simulink model "EXP1"  (R2020b)
settings: Solver=VariableStepAuto  StartTime=0.0  StopTime=200  RelTol=1e-3
settings Model: Creator=dssan  LastModifiedBy=dssan

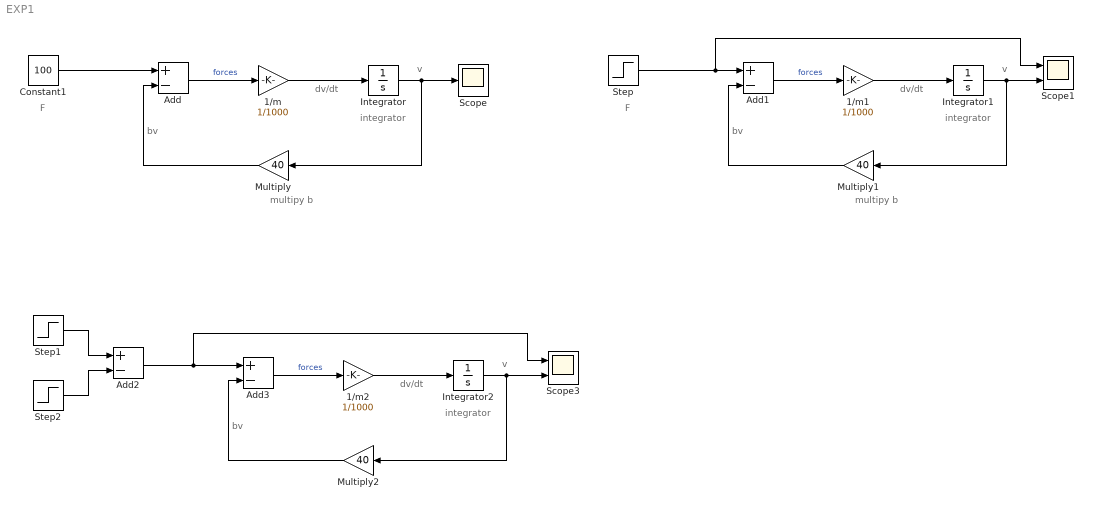
== system EXP1 ==
  note: dv/dt
  note: bv
  note: F
  note: v
  note: multipy b
  note: integrator
  note: bv
  note: v
  note: multipy b
  note: dv/dt
  note: integrator
  note: F
  note: bv
  note: v
  note: dv/dt
  note: integrator
  1/m : Gain  Gain=1/1000
  1/m1 : Gain  Gain=1/1000
  1/m2 : Gain  Gain=1/1000
  Add{,1..3} (4 alike) : Sum  Inputs=+-
  Constant1 : Constant  Value=100
  Integrator : Integrator
  Integrator1 : Integrator
  Integrator2 : Integrator
  Multiply : Gain  Gain=40
  Multiply1 : Gain  Gain=40
  Multiply2 : Gain  Gain=40
  Scope : Scope
  Scope1 : Scope  NumInputPorts=2
  Scope3 : Scope  NumInputPorts=2
  Step : Step  After=100  SampleTime=0
  Step1 : Step  Time=5  After=50  SampleTime=0
  Step2 : Step  Time=10  After=50  SampleTime=0
  wires:
  Constant1/1 -> Add/1
  Integrator/1 -> Multiply/1, Scope/1
  1/m/1 -> Integrator/1
  Add/1 -> 1/m/1  "forces"
  Multiply/1 -> Add/2
  Multiply1/1 -> Add1/2
  Add1/1 -> 1/m1/1  "forces"
  1/m1/1 -> Integrator1/1
  Integrator1/1 -> Scope1/2, Multiply1/1
  Step/1 -> Scope1/1, Add1/1
  Step1/1 -> Add2/1
  Step2/1 -> Add2/2
  Multiply2/1 -> Add3/2
  Add3/1 -> 1/m2/1  "forces"
  1/m2/1 -> Integrator2/1
  Integrator2/1 -> Scope3/2, Multiply2/1
  Add2/1 -> Scope3/1, Add3/1
